simulink model "c71_car0_template"  (R2025a)
settings: Solver=FixedStepDiscrete  StartTime=0.0  StopTime=inf  FixedStep=P_dt  RelTol=1e-3
model workspace (MAT data in the model file):
  SL_ROS_VariableLengthArrays_MaxSizes.CommonInfo.ArrayTruncateAction = 'DoNothing'
  SL_ROS_VariableLengthArrays_MaxSizes.MsgTypeMap = containers.Map
  SL_ROS_VariableLengthArrays_MaxSizes.MsgTypeMap.serialization.keys = {'mbmadmsgs/CarObsList', 'mbmadmsgs/CarOutputsExtList', 'mbmadmsgs/DriveManeuver', 'mbsafemsgs/CheckpointSequence'}
  SL_ROS_VariableLengthArrays_MaxSizes.MsgTypeMap.serialization.values{1}.PropertyName = 'list'
  SL_ROS_VariableLengthArrays_MaxSizes.MsgTypeMap.serialization.values{1}.DataType = 'mbmadmsgs/CarObs'
  SL_ROS_VariableLengthArrays_MaxSizes.MsgTypeMap.serialization.values{1}.MaxLength = 4
  SL_ROS_VariableLengthArrays_MaxSizes.MsgTypeMap.serialization.values{2}.PropertyName = 'list'
  SL_ROS_VariableLengthArrays_MaxSizes.MsgTypeMap.serialization.values{2}.DataType = 'mbmadmsgs/CarOutputsExt'
  SL_ROS_VariableLengthArrays_MaxSizes.MsgTypeMap.serialization.values{2}.MaxLength = 2
  SL_ROS_VariableLengthArrays_MaxSizes.MsgTypeMap.serialization.values{3}(1).PropertyName = 'breaks'
  SL_ROS_VariableLengthArrays_MaxSizes.MsgTypeMap.serialization.values{3}(1).DataType = 'single'
  SL_ROS_VariableLengthArrays_MaxSizes.MsgTypeMap.serialization.values{3}(1).MaxLength = 200
  SL_ROS_VariableLengthArrays_MaxSizes.MsgTypeMap.serialization.values{3}(2).PropertyName = 's1'
  SL_ROS_VariableLengthArrays_MaxSizes.MsgTypeMap.serialization.values{3}(2).DataType = 'single'
  SL_ROS_VariableLengthArrays_MaxSizes.MsgTypeMap.serialization.values{3}(2).MaxLength = 200
  SL_ROS_VariableLengthArrays_MaxSizes.MsgTypeMap.serialization.values{3}(3).PropertyName = 's2'
  SL_ROS_VariableLengthArrays_MaxSizes.MsgTypeMap.serialization.values{3}(3).DataType = 'single'
  SL_ROS_VariableLengthArrays_MaxSizes.MsgTypeMap.serialization.values{3}(3).MaxLength = 200
  SL_ROS_VariableLengthArrays_MaxSizes.MsgTypeMap.serialization.values{3}(4).PropertyName = 'segments'
  SL_ROS_VariableLengthArrays_MaxSizes.MsgTypeMap.serialization.values{3}(4).DataType = 'uint32'
  SL_ROS_VariableLengthArrays_MaxSizes.MsgTypeMap.serialization.values{3}(4).MaxLength = 200
  SL_ROS_VariableLengthArrays_MaxSizes.MsgTypeMap.serialization.values{3}(5).PropertyName = 'spline_coefs1'
  SL_ROS_VariableLengthArrays_MaxSizes.MsgTypeMap.serialization.values{3}(5).DataType = 'single'
  SL_ROS_VariableLengthArrays_MaxSizes.MsgTypeMap.serialization.values{3}(5).MaxLength = 800
  SL_ROS_VariableLengthArrays_MaxSizes.MsgTypeMap.serialization.values{3}(6).PropertyName = 'spline_coefs2'
  SL_ROS_VariableLengthArrays_MaxSizes.MsgTypeMap.serialization.values{3}(6).DataType = 'single'
  SL_ROS_VariableLengthArrays_MaxSizes.MsgTypeMap.serialization.values{3}(6).MaxLength = 800
  SL_ROS_VariableLengthArrays_MaxSizes.MsgTypeMap.serialization.values{4}.PropertyName = 'cpseq'
  SL_ROS_VariableLengthArrays_MaxSizes.MsgTypeMap.serialization.values{4}.DataType = 'mbsafemsgs/Checkpoint'
  SL_ROS_VariableLengthArrays_MaxSizes.MsgTypeMap.serialization.values{4}.MaxLength = 23
  SL_ROS_VariableLengthArrays_MaxSizes.MsgTypeMap.serialization.uniformity = 0
  SL_ROS_VariableLengthArrays_MaxSizes.MsgTypeMap.serialization.keyType = 'char'
  SL_ROS_VariableLengthArrays_MaxSizes.MsgTypeMap.serialization.valueType = 'any'
values from neighbouring files (symbols this model uses):
  CarInputsCmdForward = uint8(1)    [i01_data.m]
  CarInputsCmdHalt = uint8(0)    [i01_data.m]
  P_cpseq = Simulink.Bus.createMATLABStruct('CHECKPOINTSEQUENCEMSG', [])    [i01_data.m]
  P_display_dt = 50e-3    (= 0.05)    [s06_data.m]
  P_dt = 25e-3    (= 0.025)    [s06_data.m]
  P_p_deltan_max = 1    [d01_data.m]    (also in d71_data.m = 0.93)
  P_p_deltan_min = -P_p_deltan_max    (= -1)    [d01_data.m]    (also in d71_data.m = -0.93)
  P_p_un_max = 1    [d01_data.m]    (also in d71_data.m = 0.2)
  P_p_un_min = -P_p_un_max    (= -1)    [d01_data.m]    (also in d71_data.m = -0.2)
undefined symbols (not defined in the file or in its folder): carid, cmd, cpseq, pedals, steering
libraries: ros2lib x5, mbrt_lib_level1 x2, vrlib x1
settings Model: Creator=frank  LastModifiedBy=traenkle
settings OptimizationCC: EnhancedBackFolding=on  PassReuseOutputArgsAs=Individual arguments  ZeroExternalMemoryAtStartup=off  ZeroInternalMemoryAtStartup=off  MaxStackSize=64  OptimizeBlockOrder=speed  DifferentSizesBufferReuse=on  OptimizationCustomize=off  EfficientTunableParamExpr=on
settings DebuggingCC: ParameterTunabilityLossMsg=error  UnconnectedInputMsg=warning  UnconnectedOutputMsg=warning  UnconnectedLineMsg=warning  BusObjectLabelMismatch=error
settings HardwareCC: ProdBitPerLong=64.0  ProdHWDeviceType=Intel->x86-64 (Linux 64)
settings ModelReferenceCC: EnableRefExpFcnMdlSchedulingChecks=on
settings SFSimCC: MATLABDynamicMemAlloc=off
settings RTWCC: SystemTargetFile=ert.tlc  HardwareBoard=Robot Operating System 2 (ROS 2)  GenCodeOnly=on  TemplateMakefile=ert_default_tmf  GenerateReport=on  Toolchain=Colcon Tools  BuildConfiguration=Faster Runs  IncludeHyperlinkInReport=on  TargetLang=C++  GenerateTraceInfo=on  GPUComputeCapability=3.5  DLArmComputeVersion=19.05  Description=Embedded Coder
settings CodeAppCC: ForceParamTrailComments=on  IgnoreCustomStorageClasses=off  OperatorAnnotations=on  SimulinkDataObjDesc=on  SFDataObjDesc=on  InsertBlockDesc=on
settings ERTTargetCC: ExtModeTransport=2.0  ExtModeAutomaticAllocSize=off  InlinedParameterPlacement=Hierarchical  RootIOFormat=Structure reference  DynamicArrayContainerType=coder::array  CodeInterfacePackaging=C++ class  SubcomponentCodeInterfacePackaging=C++ class  SupportNonInlinedSFcns=on  SupportVariableSizeSignals=on

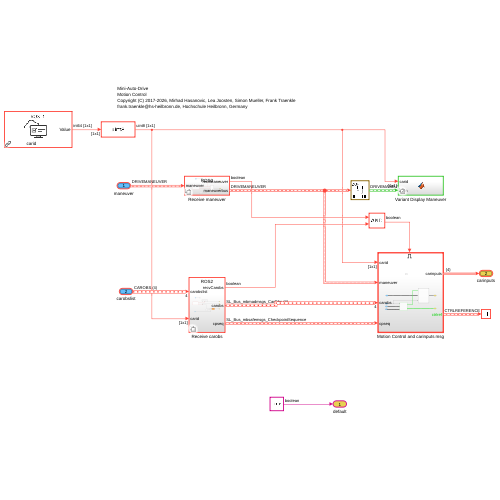
[thumbnail: Simulink's stored preview of the top-level diagram]
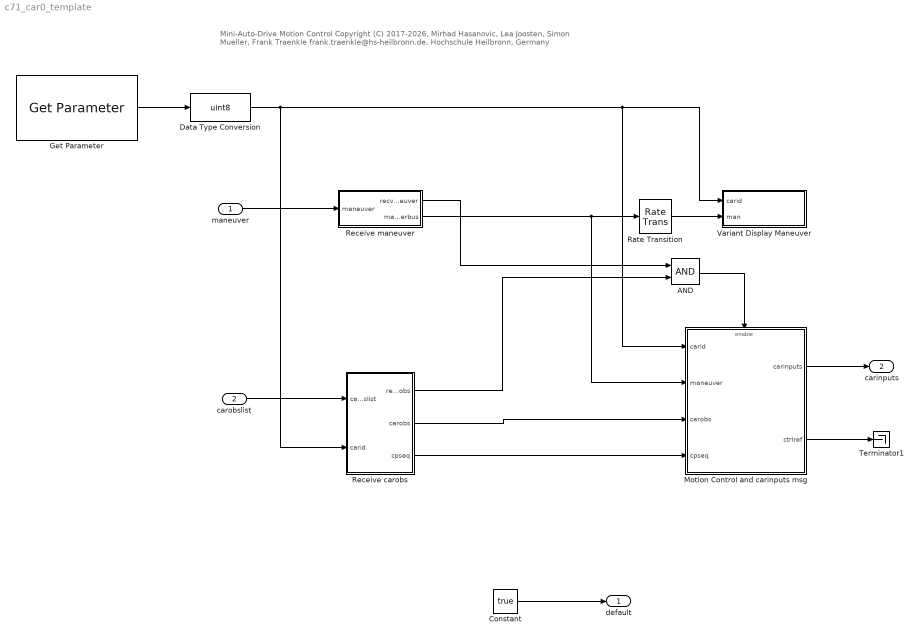
== system c71_car0_template ==
  note: Mini-Auto-Drive
      | Motion Control
      | Copyright (C) 2017-2026, Mirhad Hasanovic, Lea Joosten, Simon Mueller, Frank Traenkle
      | frank.traenkle@hs-heilbronn.de, Hochschule Heilbronn, Germany
  maneuver : Inport  OutDataTypeStr=Bus: DRIVEMANEUVER  BusOutputAsStruct=on
  carobslist : Inport  Port=2  OutDataTypeStr=Bus: CAROBS  PortDimensions=P_car_cnt  BusOutputAsStruct=on
  AND : Logic  AllPortsSameDT=off  OutDataTypeStr=boolean
  Constant : Constant  Value=true
  Data Type Conversion : DataTypeConversion  OutDataTypeStr=uint8  SaturateOnIntegerOverflow=off  RndMeth=Floor
  Get Parameter : ros2lib/Get Parameter  ParameterName=carid  ParameterType=int64  ParameterMaxArrayLength=16  ParameterInitialValue=0  SampleTime=-1  ModelName=c71_car0_template  BlockId=ParamGet_c71_car0_template_2057
  Motion Control and carinputs msg : Subsystem
  Rate Transition : RateTransition
  Receive carobs : Subsystem  Variant=on
  Receive maneuver : Subsystem  Variant=on
  Terminator1 : Terminator
  Variant Display Maneuver : Subsystem  Variant=on  VariantControlMode=sim codegen switching
  default : Outport  BusOutputAsStruct=on
  carinputs : Outport  Port=2  OutDataTypeStr=Bus: CARINPUTS  BusOutputAsStruct=on
  wires:
  Receive maneuver/1(recvManeuver) -> AND/1
  Motion Control and carinputs msg/1(carinputs) -> carinputs/1
  Receive maneuver/2(maneuverbus) -> Motion Control and carinputs msg/2(maneuver), Rate Transition/1
  Motion Control and carinputs msg/2(ctrlref) -> Terminator1/1
  Rate Transition/1 -> Variant Display Maneuver/2(man)
  maneuver/1 -> Receive maneuver/1(maneuver)
  Receive carobs/2(carobs) -> Motion Control and carinputs msg/3(carobs)
  Data Type Conversion/1 -> Receive carobs/2(carid), Motion Control and carinputs msg/1(carid), Variant Display Maneuver/1(carid)
  Receive carobs/3(cpseq) -> Motion Control and carinputs msg/4(cpseq)
  AND/1 -> Motion Control and carinputs msg/Enable
  Receive carobs/1(recvCarobs) -> AND/2
  carobslist/1 -> Receive carobs/1(carobslist)
  Constant/1 -> default/1
  Get Parameter/1 -> Data Type Conversion/1

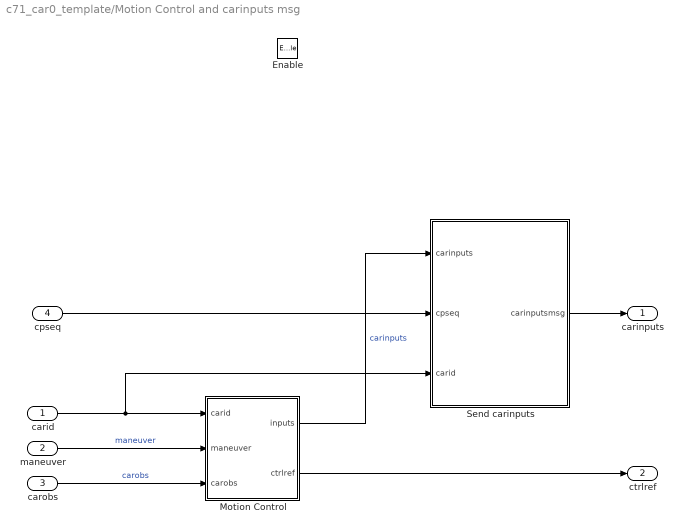
== system c71_car0_template/Motion Control and carinputs msg ==
  carid : Inport
  maneuver : Inport  Port=2
  carobs : Inport  Port=3
  cpseq : Inport  Port=4
  Enable : EnablePort
  Motion Control : Subsystem  TreatAsAtomicUnit=on  SystemSampleTime=P_dt
  Send carinputs : Subsystem  Variant=on
  carinputs : Outport
  ctrlref : Outport  Port=2
  wires:
  Send carinputs/1(carinputsmsg) -> carinputs/1
  carid/1 -> Motion Control/1(carid), Send carinputs/3(carid)
  cpseq/1 -> Send carinputs/2(cpseq)
  Motion Control/1(inputs) -> Send carinputs/1(carinputs)  "carinputs"
  Motion Control/2(ctrlref) -> ctrlref/1
  carobs/1 -> Motion Control/3(carobs)  "carobs"
  maneuver/1 -> Motion Control/2(maneuver)  "maneuver"

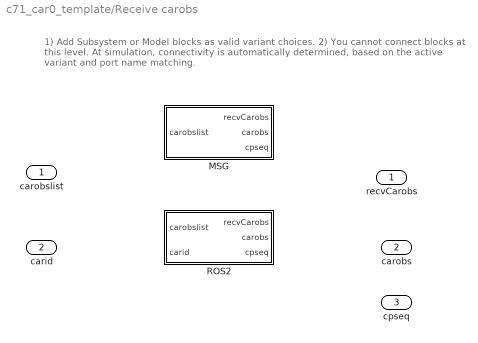
== system c71_car0_template/Receive carobs ==
  note: 1) Add Subsystem or Model blocks as valid variant choices.
      | 2) You cannot connect blocks at this level. At simulation, connectivity is automatically
      | determined, based on the active variant and port name matching.
  carobslist : Inport
  carid : Inport  Port=2
  MSG : Subsystem  VariantControl=VariantCom == VARIANT_COM_TYPE.MSG
  ROS2 : Subsystem  VariantControl=VariantCom == VARIANT_COM_TYPE.ROS2
  recvCarobs : Outport
  carobs : Outport  Port=2
  cpseq : Outport  Port=3

== system c71_car0_template/Receive maneuver ==
  note: 1) Add Subsystem or Model blocks as valid variant choices.
      | 2) You cannot connect blocks at this level. At simulation, connectivity is automatically
      | determined, based on the active variant and port name matching.
  maneuver : Inport
  MSG : Subsystem  VariantControl=VariantCom == VARIANT_COM_TYPE.MSG
  ROS2 : Subsystem  VariantControl=VariantCom == VARIANT_COM_TYPE.ROS2
  recvManeuver : Outport
  maneuverbus : Outport  Port=2

== system c71_car0_template/Variant Display Maneuver ==
  note: 1) Add Subsystem or Model blocks as valid variant choices.
      | 2) You cannot connect blocks at this level. At simulation, connectivity is automatically
      | determined, based on the active variant and port name matching.
  carid : Inport
  man : Inport  Port=2
  DisplayManeuver : MATLAB Function  TreatAsAtomicUnit=on  SystemSampleTime=P_display_dt  VariantControl=(sim)
  None : Subsystem  VariantControl=(codegen)

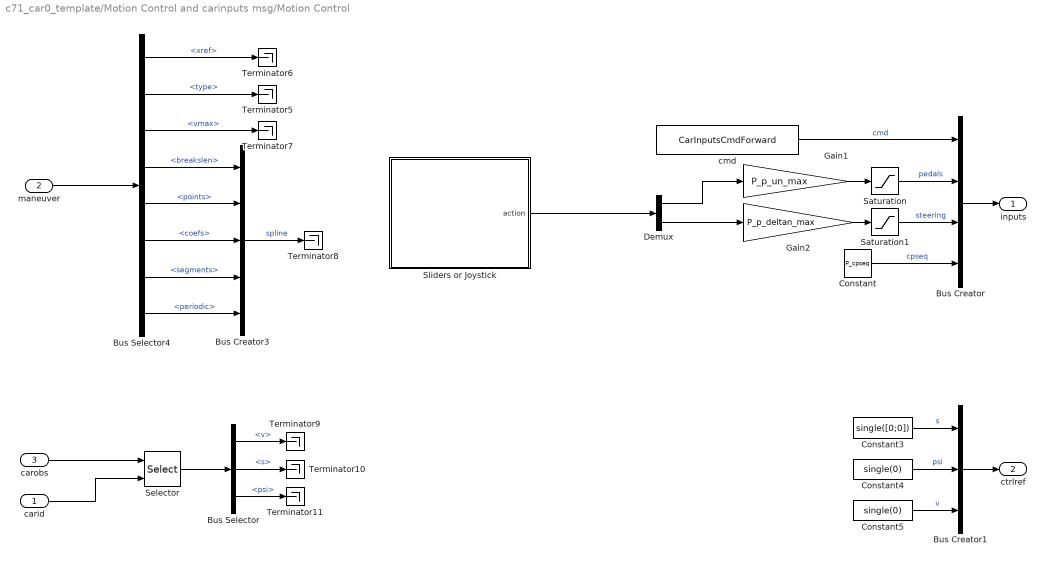
== system c71_car0_template/Motion Control and carinputs msg/Motion Control ==
  carid : Inport
  maneuver : Inport  Port=2
  carobs : Inport  Port=3
  Bus Creator : BusCreator  Inputs=4  OutDataTypeStr=Bus: CARINPUTS  NonVirtualBus=on
  Bus Creator1 : BusCreator  Inputs=3  OutDataTypeStr=Bus: CTRLREFERENCE  NonVirtualBus=on
  Bus Creator3 : BusCreator  Inputs=5  OutDataTypeStr=Bus: SPLINE
  Bus Selector : BusSelector  OutputSignals=v,s,psi
  Bus Selector4 : BusSelector  OutputSignals=xref,type,vmax,breakslen,points,coefs,segments,periodic
  Constant : Constant  Value=P_cpseq  OutDataTypeStr=Bus: CHECKPOINTSEQUENCEMSG
  Constant3 : Constant  Value=single([0;0])
  Constant4 : Constant  Value=single(0)
  Constant5 : Constant  Value=single(0)
  Demux : Demux  Outputs=2
  Gain1 : Gain  Gain=P_p_un_max
  Gain2 : Gain  Gain=P_p_deltan_max
  Saturation : Saturate  UpperLimit=P_p_un_max  LowerLimit=P_p_un_min
  Saturation1 : Saturate  UpperLimit=P_p_deltan_max  LowerLimit=P_p_deltan_min
  Selector : Selector  IndexMode=Zero-based  InputPortWidth=P_car_cnt  IndexOptions=Index vector (port)  Indices=0  OutputSizes=1
  Sliders or Joystick : Subsystem  Variant=on  VariantControlMode=label  LabelModeActiveChoice=true
  Terminator{5..11} (7 alike) : Terminator
  cmd : Constant  Value=CarInputsCmdForward
  inputs : Outport  VectorParamsAs1DForOutWhenUnconnected=off
  ctrlref : Outport  Port=2  VectorParamsAs1DForOutWhenUnconnected=off
  wires:
  Constant5/1 -> Bus Creator1/3  "v"
  Constant3/1 -> Bus Creator1/1  "s"
  Constant4/1 -> Bus Creator1/2  "psi"
  Bus Creator1/1 -> ctrlref/1
  Constant/1 -> Bus Creator/4  "cpseq"
  Demux/2 -> Gain2/1
  Demux/1 -> Gain1/1
  Sliders or Joystick/1(action) -> Demux/1
  Bus Creator/1 -> inputs/1
  Saturation/1 -> Bus Creator/2  "pedals"
  Saturation1/1 -> Bus Creator/3  "steering"
  cmd/1 -> Bus Creator/1  "cmd"
  Gain2/1 -> Saturation1/1
  Gain1/1 -> Saturation/1
  Bus Selector/2 -> Terminator10/1  "<s>"
  carobs/1 -> Selector/1
  Bus Selector/1 -> Terminator9/1  "<v>"
  Bus Selector/3 -> Terminator11/1  "<psi>"
  Selector/1 -> Bus Selector/1
  carid/1 -> Selector/2
  Bus Selector4/7 -> Bus Creator3/4  "<segments>"
  Bus Selector4/2 -> Terminator5/1  "<type>"
  maneuver/1 -> Bus Selector4/1
  Bus Selector4/3 -> Terminator7/1  "<vmax>"
  Bus Selector4/8 -> Bus Creator3/5  "<periodic>"
  Bus Creator3/1 -> Terminator8/1  "spline"
  Bus Selector4/1 -> Terminator6/1  "<xref>"
  Bus Selector4/6 -> Bus Creator3/3  "<coefs>"
  Bus Selector4/5 -> Bus Creator3/2  "<points>"
  Bus Selector4/4 -> Bus Creator3/1  "<breakslen>"

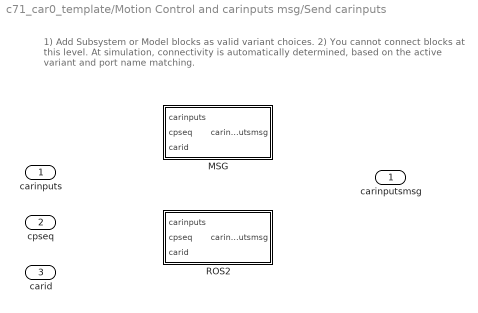
== system c71_car0_template/Motion Control and carinputs msg/Send carinputs ==
  note: 1) Add Subsystem or Model blocks as valid variant choices.
      | 2) You cannot connect blocks at this level. At simulation, connectivity is automatically
      | determined, based on the active variant and port name matching.
  carinputs : Inport
  cpseq : Inport  Port=2
  carid : Inport  Port=3
  MSG : Subsystem  VariantControl=VariantCom == VARIANT_COM_TYPE.MSG
  ROS2 : Subsystem  VariantControl=VariantCom == VARIANT_COM_TYPE.ROS2
  carinputsmsg : Outport

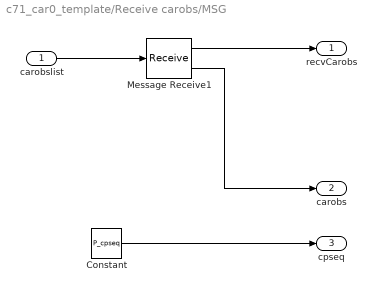
== system c71_car0_template/Receive carobs/MSG ==
  carobslist : Inport  OutDataTypeStr=Bus: CAROBS  BusOutputAsStruct=on
  Constant : Constant  Value=P_cpseq  OutDataTypeStr=Bus: CHECKPOINTSEQUENCEMSG
  Message Receive1 : Receive  InputPortMessageModes=m  UseInternalQueue=off  QueueLength=1  ShowQueueStatus=on
      settings: OutputPortMap=o0,o1
  recvCarobs : Outport
  carobs : Outport  Port=2
  cpseq : Outport  Port=3
  wires:
  Message Receive1/2 -> carobs/1
  Message Receive1/1 -> recvCarobs/1
  Constant/1 -> cpseq/1
  carobslist/1 -> Message Receive1/1

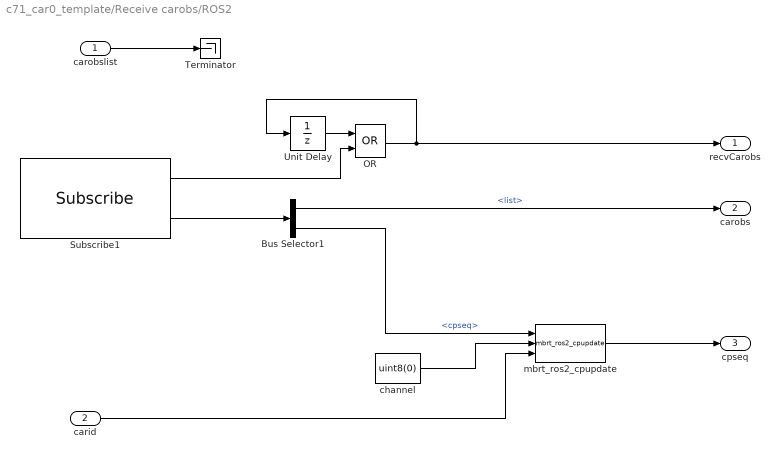
== system c71_car0_template/Receive carobs/ROS2 ==
  carobslist : Inport  OutDataTypeStr=Bus: CAROBS  BusOutputAsStruct=on
  carid : Inport  Port=2
  Bus Selector1 : BusSelector  OutputSignals=list,cpseq
  OR : Logic  Operator=OR  AllPortsSameDT=off  OutDataTypeStr=boolean
  Subscribe1 : ros2lib/Subscribe  topicSource=Specify your own  topic=/mad/locate/carobs  messageType=mbmadmsgs/CarObsList  sampleTime=-1  QOSHistory=Keep last  QOSDepth=1  QOSReliability=Best effort  QOSDurability=Volatile  QOSDeadline=Inf  QOSLifespan=Inf  QOSLiveliness=Automatic  QOSLeaseDuration=Inf  QOSAvoidROSNamespaceConventions=off
  Terminator : Terminator
  Unit Delay : UnitDelay  InitialCondition=false  SampleTime=-1  HasFrameUpgradeWarning=on
  channel : Constant  Value=uint8(0)
  mbrt_ros2_cpupdate : mbrt_lib_level1/mbrt_ros2_cpupdate  P_cur_cpid=P_cpid_CtrlStart
  recvCarobs : Outport
  carobs : Outport  Port=2
  cpseq : Outport  Port=3
  wires:
  Bus Selector1/2 -> mbrt_ros2_cpupdate/1  "<cpseq>"
  OR/1 -> recvCarobs/1, Unit Delay/1
  Subscribe1/1 -> OR/2
  Bus Selector1/1 -> carobs/1  "<list>"
  channel/1 -> mbrt_ros2_cpupdate/2
  mbrt_ros2_cpupdate/1 -> cpseq/1
  carobslist/1 -> Terminator/1
  Subscribe1/2 -> Bus Selector1/1
  Unit Delay/1 -> OR/1
  carid/1 -> mbrt_ros2_cpupdate/3

== system c71_car0_template/Receive maneuver/MSG ==
  maneuver : Inport  OutDataTypeStr=Bus: DRIVEMANEUVER  BusOutputAsStruct=on
  Message Receive : Receive  InputPortMessageModes=m  UseInternalQueue=off  QueueLength=1  ShowQueueStatus=on
      settings: OutputPortMap=o0,o1
  recvManeuver : Outport
  maneuverbus : Outport  Port=2
  wires:
  Message Receive/2 -> maneuverbus/1
  Message Receive/1 -> recvManeuver/1
  maneuver/1 -> Message Receive/1

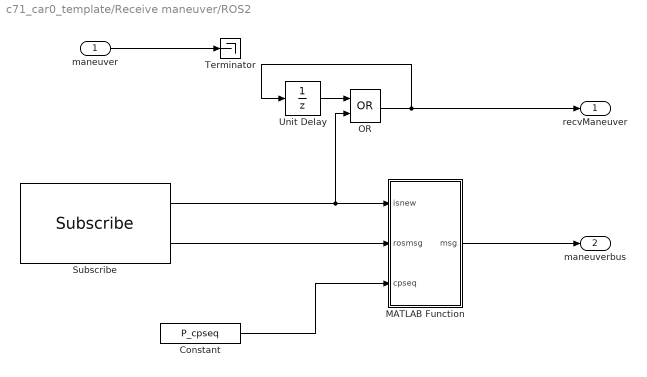
== system c71_car0_template/Receive maneuver/ROS2 ==
  maneuver : Inport  OutDataTypeStr=Bus: DRIVEMANEUVER  BusOutputAsStruct=on
  Constant : Constant  Value=P_cpseq  OutDataTypeStr=Bus: CHECKPOINTSEQUENCEMSG
  MATLAB Function : MATLAB Function  TreatAsAtomicUnit=on
  OR : Logic  Operator=OR  AllPortsSameDT=off  OutDataTypeStr=boolean
  Subscribe : ros2lib/Subscribe  topicSource=Select from ROS network  topic=/mad/car0/maneuver  messageType=mbmadmsgs/DriveManeuver  sampleTime=-1  QOSHistory=Keep last  QOSDepth=1  QOSReliability=Best effort  QOSDurability=Volatile  QOSDeadline=Inf  QOSLifespan=Inf  QOSLiveliness=Automatic  QOSLeaseDuration=Inf  QOSAvoidROSNamespaceConventions=off
  Terminator : Terminator
  Unit Delay : UnitDelay  InitialCondition=false  SampleTime=-1  HasFrameUpgradeWarning=on
  recvManeuver : Outport
  maneuverbus : Outport  Port=2
  wires:
  MATLAB Function/1(msg) -> maneuverbus/1
  maneuver/1 -> Terminator/1
  Subscribe/1 -> OR/2, MATLAB Function/1(isnew)
  Subscribe/2 -> MATLAB Function/2(rosmsg)
  Constant/1 -> MATLAB Function/3(cpseq)
  OR/1 -> recvManeuver/1, Unit Delay/1
  Unit Delay/1 -> OR/1

== system c71_car0_template/Variant Display Maneuver/None ==
  carid : Inport
  man : Inport  Port=2

== system c71_car0_template/Motion Control and carinputs msg/Motion Control/Sliders or Joystick ==
  note: 1) Add Subsystem or Model blocks as valid variant choices.
      | 2) You cannot connect blocks at this level. At simulation, connectivity is automatically
      | determined, based on the active variant and port name matching.
  Joystick : Subsystem  VariantControl=false
  Sliders : Subsystem  VariantControl=true
  action : Outport

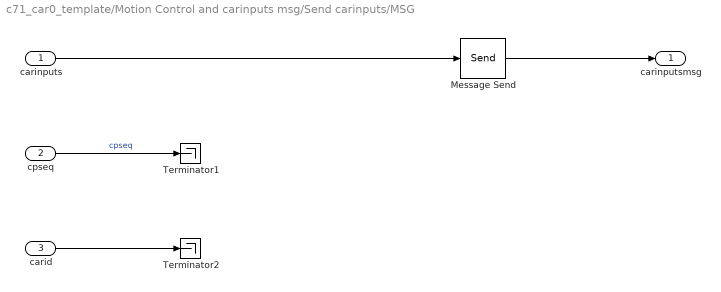
== system c71_car0_template/Motion Control and carinputs msg/Send carinputs/MSG ==
  carinputs : Inport
  cpseq : Inport  Port=2
  carid : Inport  Port=3
  Message Send : Send  OutputPortMessageModes=m
  Terminator1 : Terminator
  Terminator2 : Terminator
  carinputsmsg : Outport
  wires:
  Message Send/1 -> carinputsmsg/1
  carid/1 -> Terminator2/1
  carinputs/1 -> Message Send/1
  cpseq/1 -> Terminator1/1  "cpseq"

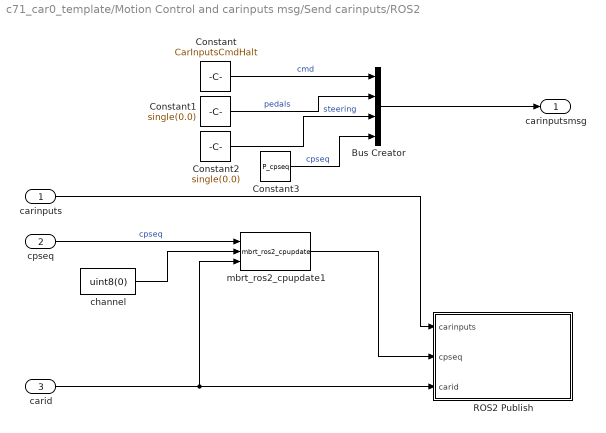
== system c71_car0_template/Motion Control and carinputs msg/Send carinputs/ROS2 ==
  carinputs : Inport
  cpseq : Inport  Port=2
  carid : Inport  Port=3
  Bus Creator : BusCreator  Inputs=4  OutDataTypeStr=Bus: CARINPUTS
  Constant : Constant  Value=CarInputsCmdHalt  SampleTime=-1
  Constant1 : Constant  Value=single(0.0)  SampleTime=-1
  Constant2 : Constant  Value=single(0.0)  SampleTime=-1
  Constant3 : Constant  Value=P_cpseq  OutDataTypeStr=Bus: CHECKPOINTSEQUENCEMSG  SampleTime=-1
  ROS2 Publish : Subsystem
  channel : Constant  Value=uint8(0)
  mbrt_ros2_cpupdate1 : mbrt_lib_level1/mbrt_ros2_cpupdate  P_cur_cpid=P_cpid_CtrlPublish
  carinputsmsg : Outport
  wires:
  carinputs/1 -> ROS2 Publish/1(carinputs)
  cpseq/1 -> mbrt_ros2_cpupdate1/1  "cpseq"
  Bus Creator/1 -> carinputsmsg/1
  mbrt_ros2_cpupdate1/1 -> ROS2 Publish/2(cpseq)
  carid/1 -> mbrt_ros2_cpupdate1/3, ROS2 Publish/3(carid)
  channel/1 -> mbrt_ros2_cpupdate1/2
  Constant/1 -> Bus Creator/1  "cmd"
  Constant1/1 -> Bus Creator/2  "pedals"
  Constant2/1 -> Bus Creator/3  "steering"
  Constant3/1 -> Bus Creator/4  "cpseq"

== system c71_car0_template/Motion Control and carinputs msg/Motion Control/Sliders or Joystick/Joystick ==
  Data Type Conversion : DataTypeConversion  OutDataTypeStr=single  SaturateOnIntegerOverflow=off  RndMeth=Floor
  Gain3 : Gain  Gain=-1
  Joystick Input : vrlib/Joystick Input  joyid=1  adjustports=off  forcefeed=off
  Selector1 : Selector  IndexOptions=Index vector (dialog)  Indices=[2 4]  OutputSizes=1
  Terminator : Terminator
  action : Outport
  wires:
  Data Type Conversion/1 -> Selector1/1
  Gain3/1 -> action/1
  Joystick Input/1 -> Data Type Conversion/1
  Selector1/1 -> Gain3/1
  Joystick Input/2 -> Terminator/1

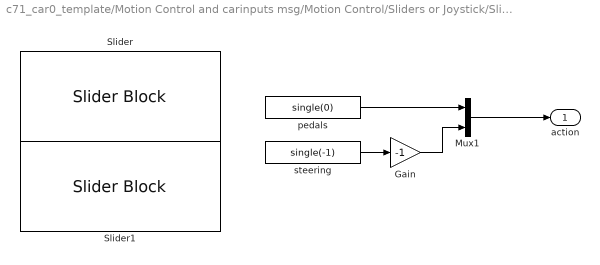
== system c71_car0_template/Motion Control and carinputs msg/Motion Control/Sliders or Joystick/Sliders ==
  Gain : Gain  Gain=-1
  Mux1 : Mux  Inputs=2
  Slider : SliderBlock  ScaleMin=-1  ScaleMax=1
  Slider1 : SliderBlock  ScaleMin=-1  ScaleMax=1
  pedals : Constant  Value=single(0)  SampleTime=Inf
  steering : Constant  Value=single(-1)
  action : Outport
  wires:
  pedals/1 -> Mux1/1
  Gain/1 -> Mux1/2
  Mux1/1 -> action/1
  steering/1 -> Gain/1

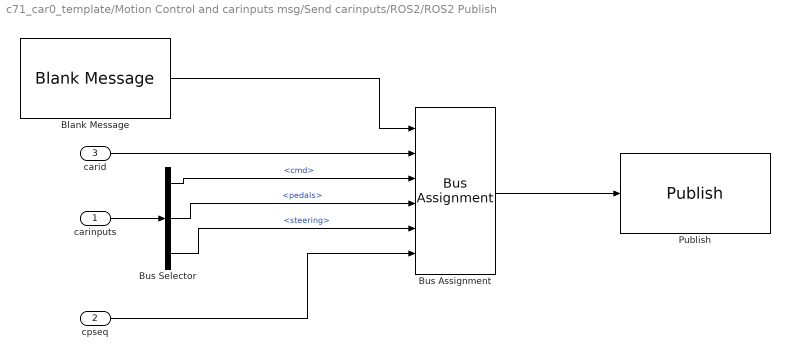
== system c71_car0_template/Motion Control and carinputs msg/Send carinputs/ROS2/ROS2 Publish ==
  carinputs : Inport
  cpseq : Inport  Port=2
  carid : Inport  Port=3
  Blank Message : ros2lib/Blank Message  messageClass=Message  entityType=mbmadmsgs/CarInputs  messageType=mbmadmsgs/CarInputs  SampleTime=inf
  Bus Assignment : BusAssignment  AssignedSignals=carid,cmd,pedals,steering,cpseq
  Bus Selector : BusSelector  OutputSignals=cmd,pedals,steering
  Publish : ros2lib/Publish  topicSource=Specify your own  topic=/mad/car0/carinputs  messageType=mbmadmsgs/CarInputs  QOSHistory=Keep last  QOSDepth=1  QOSReliability=Best effort  QOSDurability=Volatile  QOSDeadline=Inf  QOSLifespan=Inf  QOSLiveliness=Automatic  QOSLeaseDuration=Inf  QOSAvoidROSNamespaceConventions=off
  wires:
  Bus Selector/2 -> Bus Assignment/4  "<pedals>"
  Bus Selector/1 -> Bus Assignment/3  "<cmd>"
  carid/1 -> Bus Assignment/2
  Bus Selector/3 -> Bus Assignment/5  "<steering>"
  Bus Assignment/1 -> Publish/1
  carinputs/1 -> Bus Selector/1
  Blank Message/1 -> Bus Assignment/1
  cpseq/1 -> Bus Assignment/6

== matlab function c71_car0_template/Receive maneuver/ROS2/MATLAB Function ==
  data: isnew input; rosmsg input; msg output Bus: DRIVEMANEUVER; P_max_breakslen parameter uint32; cpseq input
function msg = ros2msg(isnew, rosmsg, P_max_breakslen, cpseq)
msg = struct( ...
    'vmax', rosmsg.vmax, ...
    'type', rosmsg.type, ...
    'xref', rosmsg.xref, ...
    'lapCount', rosmsg.lapcount, ...
    'disableLaneMonitor', false, ...
    'isnew', isnew, ...
    'breakslen', rosmsg.breaks_SL_Info.CurrentLength, ...
    'points', [ rosmsg.breaks' ; rosmsg.s1' ; rosmsg.s2' ], ...
    'coefs', zeros(P_max_breakslen*2, 4, 'single'), ...
    'segments', rosmsg.segments', ...
    'periodic', rosmsg.periodic, ...
    'cpseq', cpseq);
msg.coefs(1:2:end-1,:) = reshape(rosmsg.spline_coefs1, 4, P_max_breakslen)';
msg.coefs(2:2:end,:) = reshape(rosmsg.spline_coefs2, 4, P_max_breakslen)';
end

== matlab function c71_car0_template/Variant Display Maneuver/DisplayManeuver ==
  data: carid input; man input
function displayManuever(carid, man)
coder.extrinsic('line');

persistent config lineObj;

if isempty(config)
    config = mbc_config();
end

if isempty(lineObj)
    %figure(1);
    lineObj = line(man.points(2,1:man.breakslen), man.points(3,1:man.breakslen), 'Color', config.car.colors{carid+1}, 'LineStyle', '-');
end

set(lineObj, 'XData', man.points(2,1:man.breakslen), 'YData', man.points(3,1:man.breakslen));
end
